simulink model "pi_test"  (R2022b)
settings: Solver=VariableStepAuto  StartTime=0.0  StopTime=4e-8  RelTol=1e-3
libraries: dspsigops x7, msbUtilities x1
settings Model: Creator=Ali-Laptop  LastModifiedBy=Ali-Laptop

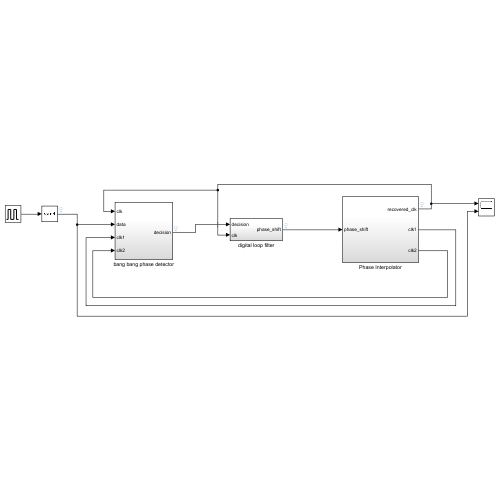
[thumbnail: Simulink's stored preview of the top-level diagram]
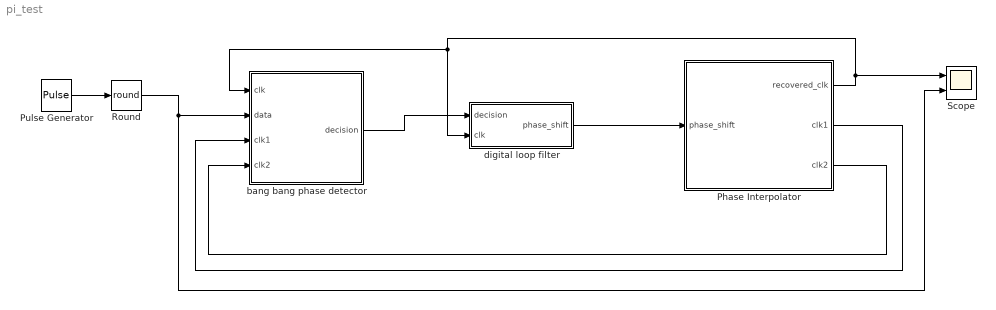
== system pi_test ==
  Phase Interpolator : Subsystem
  Pulse Generator : DiscretePulseGenerator  PulseType=Time based  Period=4e-10  PulseWidth=50  PhaseDelay=1e-10
  Round : Rounding  Operator=round
  Scope : Scope  NumInputPorts=2
  bang bang phase detector : Subsystem
  digital loop filter : Subsystem
  wires:
  digital loop filter/1(phase_shift) -> Phase Interpolator/1(phase_shift)
  Phase Interpolator/1(recovered_clk) -> digital loop filter/2(clk), bang bang phase detector/1(clk), Scope/1
  Phase Interpolator/2(clk1) -> bang bang phase detector/3(clk1)
  Phase Interpolator/3(clk2) -> bang bang phase detector/4(clk2)
  bang bang phase detector/1(decision) -> digital loop filter/1(decision)
  Round/1 -> bang bang phase detector/2(data), Scope/2
  Pulse Generator/1 -> Round/1

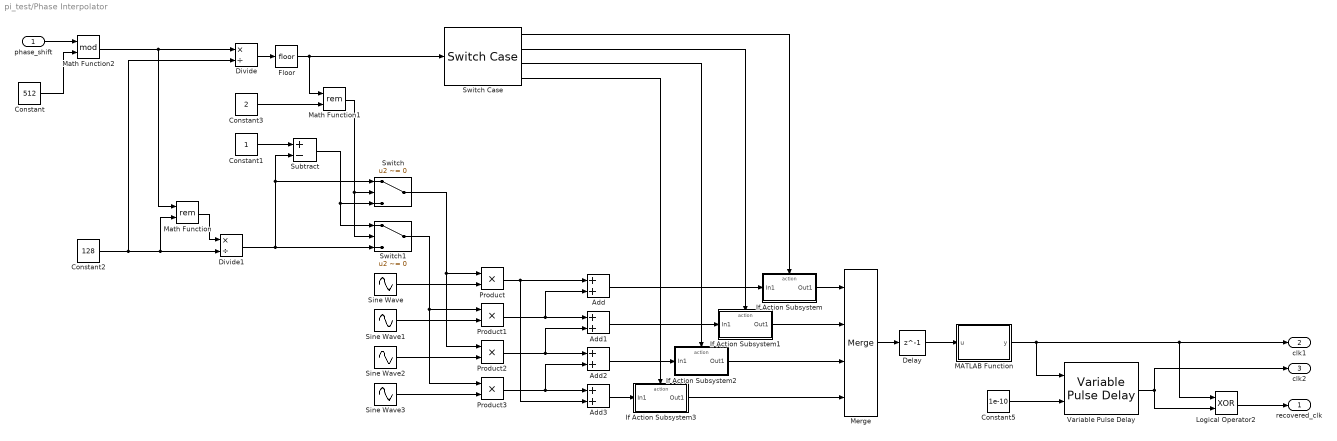
== system pi_test/Phase Interpolator ==
  phase_shift : Inport
  Add{,1..3} (4 alike) : Sum
  Constant : Constant  Value=512
  Constant1 : Constant
  Constant2 : Constant  Value=128
  Constant3 : Constant  Value=2
  Constant5 : Constant  Value=1e-10
  Delay : Delay  DelayLength=1
  Divide : Product  Inputs=*/
  Divide1 : Product  Inputs=*/
  Floor : Rounding
  If Action Subsystem : Subsystem  TreatAsAtomicUnit=on
  If Action Subsystem1 : Subsystem  TreatAsAtomicUnit=on
  If Action Subsystem2 : Subsystem  TreatAsAtomicUnit=on
  If Action Subsystem3 : Subsystem  TreatAsAtomicUnit=on
  Logical Operator2 : Logic  Operator=XOR  AllPortsSameDT=off  OutDataTypeStr=boolean
  MATLAB Function : MATLAB Function  TreatAsAtomicUnit=on
  Math Function : Math  Operator=rem
  Math Function1 : Math  Operator=rem
  Math Function2 : Math  Operator=mod
  Merge : Merge  Inputs=4
  Product{,1..3} (4 alike) : Product
  Sine Wave : Sin  Frequency=pi*5e9  SampleTime=2e-12
  Sine Wave1 : Sin  Frequency=pi*5e9  Phase=pi/2  SampleTime=2e-12
  Sine Wave2 : Sin  Frequency=pi*5e9  Phase=pi  SampleTime=2e-12
  Sine Wave3 : Sin  Frequency=pi*5e9  Phase=3*pi/2  SampleTime=2e-12
  Subtract : Sum  Inputs=+-
  Switch : Switch  Criteria=u2 ~= 0  SaturateOnIntegerOverflow=off  InputSameDT=off
  Switch Case : SwitchCase  CaseConditions={0,1,2,3}  ShowDefaultCase=off
  Switch1 : Switch  Criteria=u2 ~= 0  SaturateOnIntegerOverflow=off  InputSameDT=off
  Variable Pulse Delay : msbUtilities/Variable Pulse Delay  InitialInput=0  BufferSize=10
  recovered_clk : Outport
  clk1 : Outport  Port=2
  clk2 : Outport  Port=3
  wires:
  Switch Case/1 -> If Action Subsystem/Action
  Product/1 -> Add3/2, Add/1
  Product3/1 -> Add2/2, Add3/1
  Merge/1 -> Delay/1
  If Action Subsystem3/1(Out1) -> Merge/4
  Product1/1 -> Add1/1, Add/2
  Sine Wave3/1 -> Product3/2
  Product2/1 -> Add2/1, Add1/2
  Variable Pulse Delay/1 -> Logical Operator2/2, clk2/1
  Switch1/1 -> Product3/1, Product1/1
  Sine Wave2/1 -> Product2/2
  Constant2/1 -> Divide1/2, Math Function/2, Divide/2
  Add3/1 -> If Action Subsystem3/1(In1)
  Add/1 -> If Action Subsystem/1(In1)
  Switch/1 -> Product2/1, Product/1
  Switch Case/4 -> If Action Subsystem3/Action
  Subtract/1 -> Switch1/1, Switch/3
  Divide1/1 -> Switch/1, Subtract/2, Switch1/3
  Math Function2/1 -> Math Function/1, Divide/1
  Constant1/1 -> Subtract/1
  Math Function1/1 -> Switch1/2, Switch/2
  If Action Subsystem/1(Out1) -> Merge/1
  Divide/1 -> Floor/1
  Constant5/1 -> Variable Pulse Delay/2
  Switch Case/3 -> If Action Subsystem2/Action
  Constant3/1 -> Math Function1/2
  Switch Case/2 -> If Action Subsystem1/Action
  Sine Wave1/1 -> Product1/2
  Floor/1 -> Switch Case/1, Math Function1/1
  Logical Operator2/1 -> recovered_clk/1
  MATLAB Function/1(y) -> Variable Pulse Delay/1, clk1/1, Logical Operator2/1
  Add1/1 -> If Action Subsystem1/1(In1)
  If Action Subsystem1/1(Out1) -> Merge/2
  Sine Wave/1 -> Product/2
  Add2/1 -> If Action Subsystem2/1(In1)
  If Action Subsystem2/1(Out1) -> Merge/3
  Math Function/1 -> Divide1/1
  Delay/1 -> MATLAB Function/1(u)
  phase_shift/1 -> Math Function2/1
  Constant/1 -> Math Function2/2

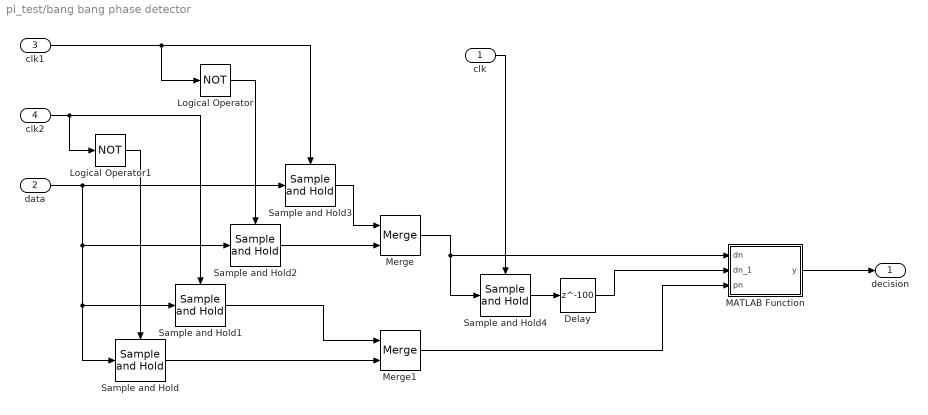
== system pi_test/bang bang phase detector ==
  clk : Inport
  data : Inport  Port=2
  clk1 : Inport  Port=3
  clk2 : Inport  Port=4
  Delay : Delay  DelayLength=100
  Logical Operator : Logic  Operator=NOT  AllPortsSameDT=off  OutDataTypeStr=boolean
  Logical Operator1 : Logic  Operator=NOT  AllPortsSameDT=off  OutDataTypeStr=boolean
  MATLAB Function : MATLAB Function  TreatAsAtomicUnit=on
  Merge : Merge
  Merge1 : Merge
  Sample and Hold{,1..4} (5 alike) : dspsigops/Sample and Hold  trig=Rising edge  initCond=0  latchinput=off
  decision : Outport
  wires:
  clk1/1 -> Sample and Hold3/Trigger, Logical Operator/1
  clk2/1 -> Logical Operator1/1, Sample and Hold1/Trigger
  data/1 -> Sample and Hold3/1, Sample and Hold1/1, Sample and Hold/1, Sample and Hold2/1
  Sample and Hold3/1 -> Merge/1
  Sample and Hold2/1 -> Merge/2
  Sample and Hold/1 -> Merge1/2
  Sample and Hold1/1 -> Merge1/1
  Merge1/1 -> MATLAB Function/3(pn)
  Sample and Hold4/1 -> Delay/1
  Merge/1 -> MATLAB Function/1(dn), Sample and Hold4/1
  MATLAB Function/1(y) -> decision/1
  clk/1 -> Sample and Hold4/Trigger
  Delay/1 -> MATLAB Function/2(dn_1)
  Logical Operator/1 -> Sample and Hold2/Trigger
  Logical Operator1/1 -> Sample and Hold/Trigger

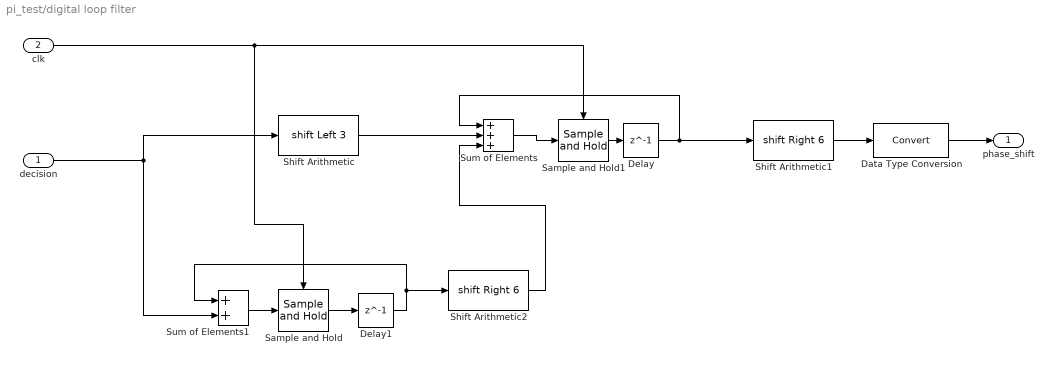
== system pi_test/digital loop filter ==
  decision : Inport
  clk : Inport  Port=2
  Data Type Conversion : DataTypeConversion  SaturateOnIntegerOverflow=off  RndMeth=Floor
  Delay : Delay  DelayLength=1
  Delay1 : Delay  DelayLength=1
  Sample and Hold : dspsigops/Sample and Hold  trig=Rising edge  initCond=0  latchinput=off
  Sample and Hold1 : dspsigops/Sample and Hold  trig=Rising edge  initCond=0  latchinput=off
  Shift Arithmetic : ArithShift  BitShiftNumber=3  BitShiftDirection=Left
  Shift Arithmetic1 : ArithShift  BitShiftNumber=6  BitShiftDirection=Right
  Shift Arithmetic2 : ArithShift  BitShiftNumber=6  BitShiftDirection=Right
  Sum of Elements : Sum  Inputs=+++
  Sum of Elements1 : Sum
  phase_shift : Outport
  wires:
  decision/1 -> Shift Arithmetic/1, Sum of Elements1/2
  Shift Arithmetic2/1 -> Sum of Elements/3
  Delay1/1 -> Sum of Elements1/1, Shift Arithmetic2/1
  Shift Arithmetic/1 -> Sum of Elements/2
  Delay/1 -> Shift Arithmetic1/1, Sum of Elements/1
  Sum of Elements1/1 -> Sample and Hold/1
  Sum of Elements/1 -> Sample and Hold1/1
  Shift Arithmetic1/1 -> Data Type Conversion/1
  clk/1 -> Sample and Hold1/Trigger, Sample and Hold/Trigger
  Sample and Hold1/1 -> Delay/1
  Sample and Hold/1 -> Delay1/1
  Data Type Conversion/1 -> phase_shift/1

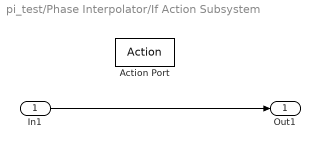
== system pi_test/Phase Interpolator/If Action Subsystem ==
  In1 : Inport
  Action Port : ActionPort  ActionPortLabel=case [ 0 ]:
  Out1 : Outport
  wires:
  In1/1 -> Out1/1

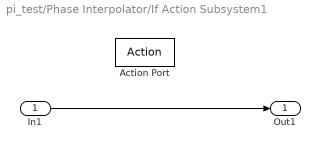
== system pi_test/Phase Interpolator/If Action Subsystem1 ==
  In1 : Inport
  Action Port : ActionPort  ActionPortLabel=case [ 1 ]:
  Out1 : Outport
  wires:
  In1/1 -> Out1/1

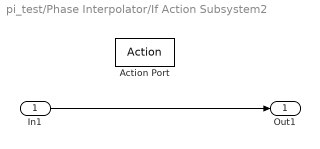
== system pi_test/Phase Interpolator/If Action Subsystem2 ==
  In1 : Inport
  Action Port : ActionPort  ActionPortLabel=case [ 2 ]:
  Out1 : Outport
  wires:
  In1/1 -> Out1/1

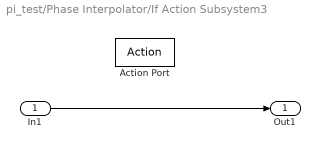
== system pi_test/Phase Interpolator/If Action Subsystem3 ==
  In1 : Inport
  Action Port : ActionPort  ActionPortLabel=case [ 3 ]:
  Out1 : Outport
  wires:
  In1/1 -> Out1/1

== matlab function pi_test/Phase Interpolator/MATLAB Function ==
  data: u input; y output
function y = fcn(u)
if u > 0
    y = 1;
else
    y = 0;
end

== matlab function pi_test/bang bang phase detector/MATLAB Function ==
  data: dn input; dn_1 input; y output; pn input
function y = fcn(dn, dn_1, pn)

y = 0;
if dn == dn_1
    y = 0;
elseif pn == dn
    y = 1;
elseif pn == dn_1
    y = -1;
end
